simulink model "CPS_unforced_s_space"  (R2022b)
settings: Solver=VariableStepAuto  StartTime=0.0  StopTime=10.0  RelTol=1e-3
values from neighbouring files (symbols this model uses):
  c = 2*dampratio*sqrt(k*M)    [CPS_sims_and_analysis.m]    (also in command_limits_check.m; ringdown-circcyl-M10-d0_001-F1-workspace.mat = 0.125663706144; setup_CPS_parameters.m)
  k = (2*pi*f_nat)^2*M    (= 394.784176044)    [CPS_sims_and_analysis.m]    (also in command_limits_check.m = 98.6960440109; ringdown-circcyl-M10-d0_001-F1-workspace.mat; setup_CPS_parameters.m = 98.6960440109)
  M = 10    [CPS_sims_and_analysis.m]    (also in command_limits_check.m; ringdown-circcyl-M10-d0_001-F1-workspace.mat; setup_CPS_parameters.m)
  T = 0.0002    [ringdown-circcyl-M10-d0_001-F1-workspace.mat]    (also in setup_CPS_parameters.m = 0.001)
  x_0 = 5    [CPS_error.m]    (also in analytical_solution_cps.m)
settings Model: Creator=eericks1  LastModifiedBy=eericks1

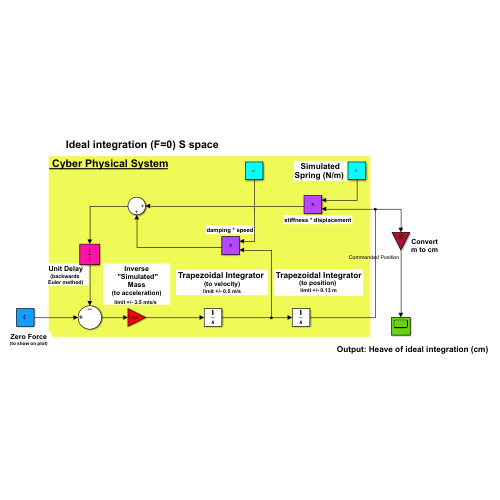
[thumbnail: Simulink's stored preview of the top-level diagram]
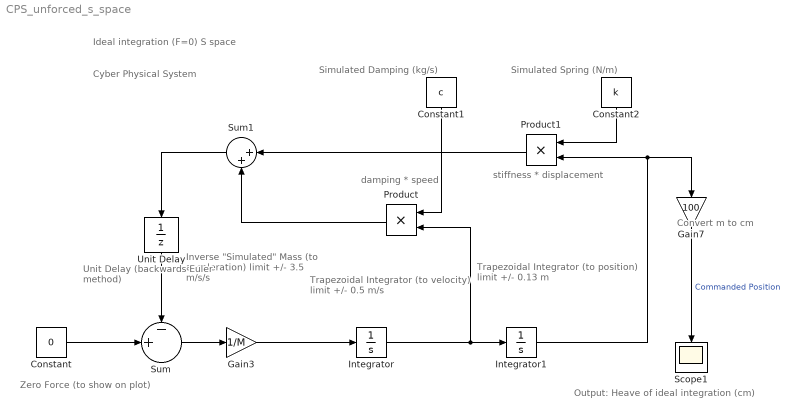
== system CPS_unforced_s_space ==
  note: stiffness * displacement
  note: Inverse
      | "Simulated"
      | Mass
      | (to acceleration)
      | limit +/- 3.5 m/s/s
  note: damping * speed
  note: Trapezoidal Integrator
      | (to velocity)
      | limit +/- 0.5 m/s
  note: Unit Delay
      | (backwards
      | Euler method)
  note: Simulated
      | Spring (N/m)
  note: Convert
      | m to cm
  note: Zero Force
      | (to show on plot)
  note: Trapezoidal Integrator
      | (to position)
      | limit +/- 0.13 m
  note: Cyber Physical System
  note: Output: Heave of ideal integration (cm)
  note: Simulated
      | Damping (kg/s)
  note: Ideal integration (F=0) S space
  Constant : Constant  Value=0  SampleTime=T
  Constant1 : Constant  Value=c  SampleTime=T
  Constant2 : Constant  Value=k  SampleTime=T
  Gain3 : Gain  Gain=1/M
  Gain7 : Gain  Gain=100
  Integrator : Integrator
  Integrator1 : Integrator
  Product : Product
  Product1 : Product
  Scope1 : Scope
  Sum : Sum  Inputs=-+|
  Sum1 : Sum  Inputs=|++
  Unit Delay : UnitDelay  InitialCondition=x_0*k/100  SampleTime=-1  HasFrameUpgradeWarning=on
  wires:
  Product/1 -> Sum1/2
  Sum1/1 -> Unit Delay/1
  Product1/1 -> Sum1/1
  Constant/1 -> Sum/2
  Sum/1 -> Gain3/1
  Constant2/1 -> Product1/1
  Unit Delay/1 -> Sum/1
  Constant1/1 -> Product/1
  Gain3/1 -> Integrator/1
  Gain7/1 -> Scope1/1  "Commanded Position"
  Integrator/1 -> Product/2, Integrator1/1
  Integrator1/1 -> Gain7/1, Product1/2
